simulink model "Lab3_22320404_375334"  (R2022a)
settings: Solver=VariableStepAuto  StartTime=0.0  StopTime=0.5  RelTol=1e-3
values from neighbouring files (symbols this model uses):
  b = 0.06    [Lab3_22320404.m]    (also in lab3.m)
  J_L = 0.00703    [Lab3_22320404.m]    (also in lab3.m)
  J_M = 0.00234    [Lab3_22320404.m]    (also in lab3.m)
  k = 350    [Lab3_22320404.m]    (also in lab3.m)
  La = 0.00035    [Lab3_22320404.m]    (also in lab3.m)
  psi = 0.28648    [Lab3_22320404.m]    (also in lab3.m)
  Ra = 0.35    [Lab3_22320404.m]    (also in lab3.m)
  U = 12    [Lab3_22320404.m]    (also in lab3.m)
libraries: fl_lib x18, nesl_utility x10, ee_lib x2, simulink x1
settings Model: Creator=90506  LastModifiedBy=81502
settings ModelReferenceCC: EnableRefExpFcnMdlSchedulingChecks=off
settings RTWCC: Description=Generic Real-Time Target  GPUComputeCapability=5.0

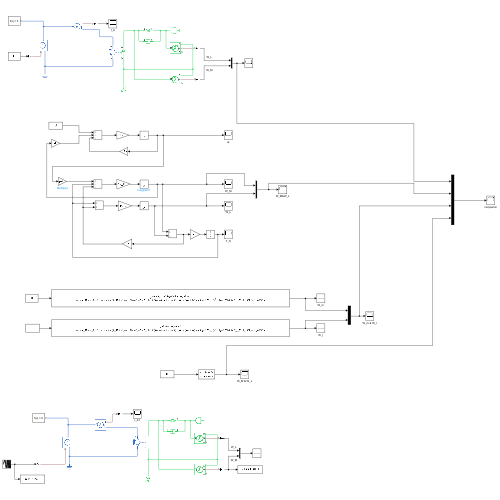
[thumbnail: Simulink's stored preview of the top-level diagram]
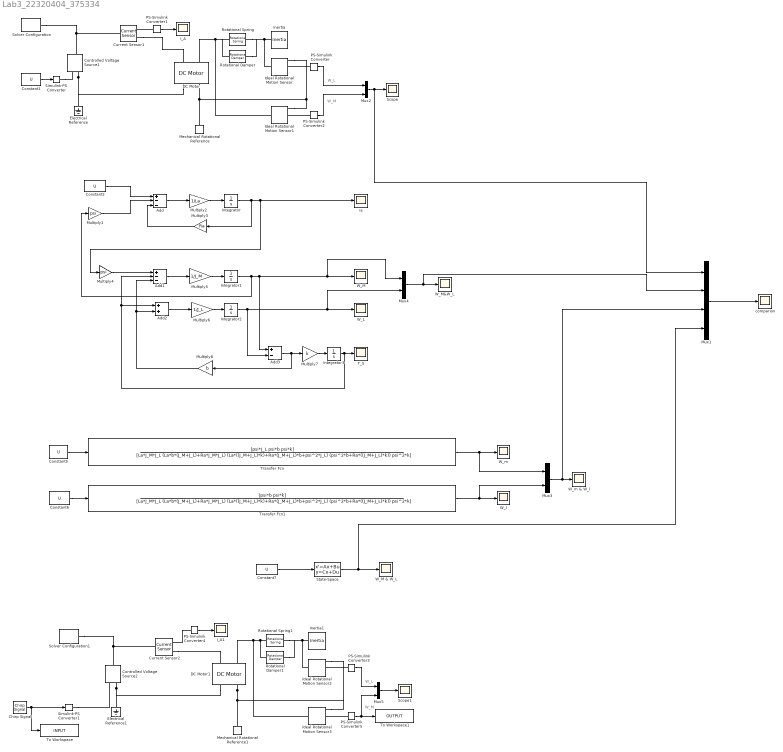
== system Lab3_22320404_375334 ==
  note: W_L
  note: W_M
  note: W_L
  note: W_M
  Add : Sum  Inputs=+--
  Add1 : Sum  Inputs=+--
  Add2 : Sum
  Add3 : Sum  Inputs=+-
  Chirp Signal : simulink/Sources/Chirp Signal  f1=0.1  T=250  f2=500
  Constant{1..2,5..7} (5 alike) : Constant  Value=U
  Controlled Voltage Source1 : fl_lib/Electrical/Electrical Sources/Controlled Voltage Source
      settings: SourceProductBaseCode=PW,SS,VE
  Controlled Voltage Source2 : fl_lib/Electrical/Electrical Sources/Controlled Voltage Source
      settings: SourceProductBaseCode=PW,SS,VE
  Current Sensor1 : fl_lib/Electrical/Electrical Sensors/Current Sensor
      settings: SourceProductBaseCode=PW,SS,VE
  Current Sensor2 : fl_lib/Electrical/Electrical Sensors/Current Sensor
      settings: SourceProductBaseCode=PW,SS,VE
  DC Motor : ee_lib/Electromechanical/Brushed Motors/DC Motor  field_option=ee.enum.field_option.pm  Rf=100 Ohm  Lf=1 H  Laf=0.15 H  If0=0 A  parameterization=ee.enum.dcparam_option.circuit_param  Ra=Ra Ohm  La=La H  emf_or_torque=ee.enum.emf_or_torque.kv  Kv=psi V*s/rad  Ki=6.876e-4 N*m/A  T_stall=0.24e-3 N*m  w_max=19100 rpm  w_rated=15000 rpm  P_rated=0.08 W  V_rated=1.5 V  lam_param=ee.enum.lam_param.damping  i_noload=0 A  V_i_noload=1.5 V  J=J_M kg*m^2  lam=0 N*m*s/rad  speed0=0 rpm  enable_fault_armature=simscape.enum.onoff.off  rev_faulted=1 / 3  G_faulted_armature=1e-5 S  fault_trigger_armature=ee.enum.faults.faultTrigger.temporal  t_fault_armature=1 s  max_permissible_current_armature=inf A  t_fail_on_current_armature=1 s  enable_fault_field=simscape.enum.onoff.off  G_faulted_field=1e-5 S  fault_trigger_field=ee.enum.faults.faultTrigger.temporal  t_fault_field=1 s  max_permissible_current_field=inf A  t_fail_on_current_field=1 s  fault_action=simscape.enum.assert.action.none  alpha=3.93e-3 1/K  Tmeas=25 degC  thermal_mass=100 J/K  initial_temperature=25 degC
  DC Motor1 : ee_lib/Electromechanical/Brushed Motors/DC Motor  field_option=ee.enum.field_option.pm  Rf=100 Ohm  Lf=1 H  Laf=0.15 H  If0=0 A  parameterization=ee.enum.dcparam_option.circuit_param  Ra=Ra Ohm  La=La H  emf_or_torque=ee.enum.emf_or_torque.kv  Kv=psi V*s/rad  Ki=6.876e-4 N*m/A  T_stall=0.24e-3 N*m  w_max=19100 rpm  w_rated=15000 rpm  P_rated=0.08 W  V_rated=1.5 V  lam_param=ee.enum.lam_param.damping  i_noload=0 A  V_i_noload=1.5 V  J=J_M kg*m^2  lam=0 N*m*s/rad  speed0=0 rpm  enable_fault_armature=simscape.enum.onoff.off  rev_faulted=1 / 3  G_faulted_armature=1e-5 S  fault_trigger_armature=ee.enum.faults.faultTrigger.temporal  t_fault_armature=1 s  max_permissible_current_armature=inf A  t_fail_on_current_armature=1 s  enable_fault_field=simscape.enum.onoff.off  G_faulted_field=1e-5 S  fault_trigger_field=ee.enum.faults.faultTrigger.temporal  t_fault_field=1 s  max_permissible_current_field=inf A  t_fail_on_current_field=1 s  fault_action=simscape.enum.assert.action.none  alpha=3.93e-3 1/K  Tmeas=25 degC  thermal_mass=100 J/K  initial_temperature=25 degC
  Electrical Reference : fl_lib/Electrical/Electrical Elements/Electrical Reference
      settings: SourceProductBaseCode=PW,SS,VE
  Electrical Reference1 : fl_lib/Electrical/Electrical Elements/Electrical Reference
      settings: SourceProductBaseCode=PW,SS,VE
  I_A : Scope
  I_A1 : Scope
  Ideal Rotational Motion Sensor{,1..3} (4 alike) : fl_lib/Mechanical/Mechanical Sensors/Ideal Rotational Motion Sensor  wrap_angle=false  offset=0 rad
      settings: SourceProductBaseCode=PW,SS,VE
  Inertia : fl_lib/Mechanical/Rotational Elements/Inertia  inertia=J_L kg*m^2  num_ports=foundation.enum.numPorts2.one  w_specify=off  w_priority=High  w=0 rad/s  w_nominal_specify=off  w_nominal_unit=rad/s  w_nominal_value=1  t_specify=off  t_priority=None  t=0 N*m  t_nominal_specify=off  t_nominal_unit=N*m  t_nominal_value=1
      settings: SourceProductBaseCode=PW,SS,VE
  Inertia1 : fl_lib/Mechanical/Rotational Elements/Inertia  inertia=J_L kg*m^2  num_ports=foundation.enum.numPorts2.one  w_specify=off  w_priority=High  w=0 rad/s  w_nominal_specify=off  w_nominal_unit=rad/s  w_nominal_value=1  t_specify=off  t_priority=None  t=0 N*m  t_nominal_specify=off  t_nominal_unit=N*m  t_nominal_value=1
      settings: SourceProductBaseCode=PW,SS,VE
  Integrator{,1..3} (4 alike) : Integrator
  Mechanical Rotational Reference : fl_lib/Mechanical/Rotational Elements/Mechanical Rotational Reference
      settings: SourceProductBaseCode=PW,SS,VE
  Mechanical Rotational Reference1 : fl_lib/Mechanical/Rotational Elements/Mechanical Rotational Reference
      settings: SourceProductBaseCode=PW,SS,VE
  Multiply1 : Gain  Gain=psi
  Multiply2 : Gain  Gain=1/La
  Multiply3 : Gain  Gain=Ra
  Multiply4 : Gain  Gain=psi
  Multiply5 : Gain  Gain=1/J_M
  Multiply6 : Gain  Gain=1/J_L
  Multiply7 : Gain  Gain=k
  Multiply8 : Gain  Gain=b
  Mux1 : Mux
  Mux{2..5} (4 alike) : Mux  Inputs=2
  PS-Simulink Converter{,1..5} (6 alike) : nesl_utility/PS-Simulink Converter  PhysicalDomain=network_engine_domain  SubClassName=ps_output  LeftPortType=input  RightPortType=output  PseudoPeriodic=off  Frequencies=[]  VectorFormat=inherit  Unit=inherit  AffineConversion=off
      settings: SourceProductBaseCode=SS,PW,VE
  Rotational Damper : fl_lib/Mechanical/Rotational Elements/Rotational Damper  D=b N*m*s/rad  w_specify=off  w_priority=None  w=0 rad/s  w_nominal_specify=off  w_nominal_unit=rad/s  w_nominal_value=1  t_specify=off  t_priority=None  t=0 N*m  t_nominal_specify=off  t_nominal_unit=N*m  t_nominal_value=1
      settings: SourceProductBaseCode=PW,SS,VE
  Rotational Damper1 : fl_lib/Mechanical/Rotational Elements/Rotational Damper  D=b N*m*s/rad  w_specify=off  w_priority=None  w=0 rad/s  w_nominal_specify=off  w_nominal_unit=rad/s  w_nominal_value=1  t_specify=off  t_priority=None  t=0 N*m  t_nominal_specify=off  t_nominal_unit=N*m  t_nominal_value=1
      settings: SourceProductBaseCode=PW,SS,VE
  Rotational Spring : fl_lib/Mechanical/Rotational Elements/Rotational Spring  spr_rate=k N*m/rad  w_specify=off  w_priority=None  w=0 rad/s  w_nominal_specify=off  w_nominal_unit=rad/s  w_nominal_value=1  t_specify=off  t_priority=None  t=0 N*m  t_nominal_specify=off  t_nominal_unit=N*m  t_nominal_value=1  phi_specify=off  phi_priority=High  phi=0 rad  phi_nominal_specify=off  phi_nominal_unit=rad  phi_nominal_value=1
      settings: SourceProductBaseCode=PW,SS,VE
  Rotational Spring1 : fl_lib/Mechanical/Rotational Elements/Rotational Spring  spr_rate=k N*m/rad  w_specify=off  w_priority=None  w=0 rad/s  w_nominal_specify=off  w_nominal_unit=rad/s  w_nominal_value=1  t_specify=off  t_priority=None  t=0 N*m  t_nominal_specify=off  t_nominal_unit=N*m  t_nominal_value=1  phi_specify=off  phi_priority=High  phi=0 rad  phi_nominal_specify=off  phi_nominal_unit=rad  phi_nominal_value=1
      settings: SourceProductBaseCode=PW,SS,VE
  Scope : Scope
  Scope1 : Scope
  Simulink-PS Converter : nesl_utility/Simulink-PS Converter  PhysicalDomain=network_engine_domain  SubClassName=ps_input  LeftPortType=input  RightPortType=output  PseudoPeriodic=off  Frequencies=[]  NoiseDistribution=none  NoiseParameters=[]  Unit=1  AffineConversion=off  FilteringAndDerivatives=provide  SimscapeFilterOrder=1  InputFilterTimeConstant=0.001  UdotUserProvided=0
      settings: SourceProductBaseCode=SS,PW,VE
  Simulink-PS Converter1 : nesl_utility/Simulink-PS Converter  PhysicalDomain=network_engine_domain  SubClassName=ps_input  LeftPortType=input  RightPortType=output  PseudoPeriodic=off  Frequencies=[]  NoiseDistribution=none  NoiseParameters=[]  Unit=1  AffineConversion=off  FilteringAndDerivatives=provide  SimscapeFilterOrder=1  InputFilterTimeConstant=0.001  UdotUserProvided=0
      settings: SourceProductBaseCode=SS,PW,VE
  Solver Configuration : nesl_utility/Solver Configuration  PhysicalDomain=network_engine_domain  SubClassName=solver  LeftPortType=input  RightPortType=generic  Tones=[]  Harmonics=[]  SimulateNoise=off  Profile=off  UseLocalSampling=off  EnableSwitchedLinearOptims=on  FrequencyDomain=off  UseCCode=off  RelTol=0.001  AbsTol=0.001  MinStep=1e-09  ToWorkspace=off  RevertToSquareIcSolve=off  NumHomotopyIterations=100  PhasorMode=off  PhasorModeNumHarmonics=1  IndexReductionMethod=DerivativeReplacement  DoDC=off  ResidualTolerance=1e-09  UseLocalSolver=off  LocalSolverChoice=NE_BACKWARD_EULER_ADVANCER  LocalSolverSampleTime=0.001  DoFixedCost=off  MaxNonlinIter=3  MaxModeIter=2  ComputeImpulses=off  ImpulseIterations=2  LinearAlgebra=auto  LinearAlgebraNumThread=0  EquationFormulation=NE_TIME_EF  DelaysMemoryBudget=1024  AutomaticFiltering=on  FilteringTimeConstant=0.001  PartitionStorageMethod=AS_NEEDED  PartitionMemoryBudget=1024  PartitionMethod=ROBUST
      settings: SourceProductBaseCode=SS,PW,VE
  Solver Configuration1 : nesl_utility/Solver Configuration  PhysicalDomain=network_engine_domain  SubClassName=solver  LeftPortType=input  RightPortType=generic  Tones=[]  Harmonics=[]  SimulateNoise=off  Profile=off  UseLocalSampling=off  EnableSwitchedLinearOptims=on  FrequencyDomain=off  UseCCode=off  RelTol=0.001  AbsTol=0.001  MinStep=1e-09  ToWorkspace=off  RevertToSquareIcSolve=off  NumHomotopyIterations=100  PhasorMode=off  PhasorModeNumHarmonics=1  IndexReductionMethod=DerivativeReplacement  DoDC=off  ResidualTolerance=1e-09  UseLocalSolver=off  LocalSolverChoice=NE_BACKWARD_EULER_ADVANCER  LocalSolverSampleTime=0.001  DoFixedCost=off  MaxNonlinIter=3  MaxModeIter=2  ComputeImpulses=off  ImpulseIterations=2  LinearAlgebra=auto  LinearAlgebraNumThread=0  EquationFormulation=NE_TIME_EF  DelaysMemoryBudget=1024  AutomaticFiltering=on  FilteringTimeConstant=0.001  PartitionStorageMethod=AS_NEEDED  PartitionMemoryBudget=1024  PartitionMethod=ROBUST
      settings: SourceProductBaseCode=SS,PW,VE
  State-Space : StateSpace  A=[-Ra/La -psi/La 0 0;psi/J_M -b/J_M b/J_M -1/J_M;0 b/J_L -b/J_L 1/J_L;0 k -k 0]  B=[1/La;0;0;0]  C=[0 1 0 0;0 0 1 0]  D=[0;0]  InitialCondition=0
  T_S : Scope
  To Workspace : ToWorkspace  VariableName=INPUT  SampleTime=0.001
  To Workspace1 : ToWorkspace  VariableName=OUTPUT  SampleTime=0.001
  Transfer Fcn : TransferFcn  Numerator=[psi*J_L psi*b psi*k]  Denominator=[La*J_M*J_L (La*b*(J_M+J_L)+Ra*J_M*J_L) (La*((J_M+J_L)*k)+Ra*(J_M+J_L)*b+psi^2*J_L) (psi^2*b+Ra*((J_M+J_L)*k)) psi^2*k]
  Transfer Fcn1 : TransferFcn  Numerator=[psi*b psi*k]  Denominator=[La*J_M*J_L (La*b*(J_M+J_L)+Ra*J_M*J_L) (La*((J_M+J_L)*k)+Ra*(J_M+J_L)*b+psi^2*J_L) (psi^2*b+Ra*((J_M+J_L)*k)) psi^2*k]
  W_L : Scope
  W_M : Scope
  W_M & W_L : Scope
  W_M&W_L : Scope
  W_l : Scope
  W_m : Scope
  W_m & W_l : Scope
  comparion : Scope
  ia : Scope
  wires:
  Constant1/1 -> Simulink-PS Converter/1
  PS-Simulink Converter1/1 -> I_A/1
  PS-Simulink Converter/1 -> Mux2/1
  PS-Simulink Converter2/1 -> Mux2/2
  Mux2/1 -> Mux1/1, Scope/1
  Add/1 -> Multiply2/1
  Multiply1/1 -> Add/2
  Multiply2/1 -> Integrator/1
  Add1/1 -> Multiply5/1
  Multiply5/1 -> Integrator1/1
  Multiply3/1 -> Add/3
  Multiply4/1 -> Add1/1
  Integrator/1 -> Multiply3/1, Multiply4/1, ia/1
  Constant2/1 -> Add/1
  Add2/1 -> Multiply6/1
  Multiply6/1 -> Integrator2/1
  Integrator2/1 -> Mux4/2, W_L/1, Add3/2
  Add3/1 -> Multiply7/1, Multiply8/1
  Multiply8/1 -> Add1/3, Add2/2
  Multiply7/1 -> Integrator3/1
  Integrator3/1 -> Add2/1, Add1/2, T_S/1
  Transfer Fcn1/1 -> W_l/1, Mux3/2
  Transfer Fcn/1 -> Mux3/1, W_m/1
  Constant6/1 -> Transfer Fcn1/1
  Constant5/1 -> Transfer Fcn/1
  Mux1/1 -> comparion/1
  State-Space/1 -> Mux1/4, W_M & W_L/1
  Constant7/1 -> State-Space/1
  Integrator1/1 -> Multiply1/1, Mux4/1, W_M/1, Add3/1
  Mux3/1 -> Mux1/3, W_m & W_l/1
  Mux4/1 -> Mux1/2, W_M&W_L/1
  Mux5/1 -> Scope1/1
  PS-Simulink Converter3/1 -> Mux5/1
  PS-Simulink Converter5/1 -> To Workspace1/1, Mux5/2
  PS-Simulink Converter4/1 -> I_A1/1
  Chirp Signal/1 -> Simulink-PS Converter1/1, To Workspace/1
  connections:
  Solver Configuration/RConn1 -- Controlled Voltage Source1/LConn1 -- Current Sensor1/LConn1
  Controlled Voltage Source1/RConn2 -- Electrical Reference/LConn1 -- DC Motor/RConn1
  Ideal Rotational Motion Sensor1/LConn1 -- Rotational Spring/LConn1 -- Rotational Damper/LConn1 -- DC Motor/LConn2
  Ideal Rotational Motion Sensor/RConn1 -- Mechanical Rotational Reference/LConn1 -- DC Motor/RConn2 -- Ideal Rotational Motion Sensor1/RConn1
  Simulink-PS Converter/RConn1 -- Controlled Voltage Source1/RConn1
  PS-Simulink Converter1/LConn1 -- Current Sensor1/RConn1
  PS-Simulink Converter/LConn1 -- Ideal Rotational Motion Sensor/RConn2
  Current Sensor1/RConn2 -- DC Motor/LConn1
  PS-Simulink Converter2/LConn1 -- Ideal Rotational Motion Sensor1/RConn2
  Ideal Rotational Motion Sensor/LConn1 -- Rotational Damper/RConn1 -- Rotational Spring/RConn1 -- Inertia/LConn1
  Controlled Voltage Source2/RConn2 -- Electrical Reference1/LConn1 -- DC Motor1/RConn1
  DC Motor1/RConn2 -- Mechanical Rotational Reference1/LConn1 -- Ideal Rotational Motion Sensor2/RConn1 -- Ideal Rotational Motion Sensor3/RConn1
  Solver Configuration1/RConn1 -- Controlled Voltage Source2/LConn1 -- Current Sensor2/LConn1
  Rotational Damper1/LConn1 -- Ideal Rotational Motion Sensor3/LConn1 -- DC Motor1/LConn2 -- Rotational Spring1/LConn1
  Ideal Rotational Motion Sensor2/LConn1 -- Rotational Damper1/RConn1 -- Rotational Spring1/RConn1 -- Inertia1/LConn1
  Simulink-PS Converter1/RConn1 -- Controlled Voltage Source2/RConn1
  PS-Simulink Converter5/LConn1 -- Ideal Rotational Motion Sensor3/RConn2
  PS-Simulink Converter4/LConn1 -- Current Sensor2/RConn1
  Current Sensor2/RConn2 -- DC Motor1/LConn1
  PS-Simulink Converter3/LConn1 -- Ideal Rotational Motion Sensor2/RConn2
